simulink model "ex1_500KV_2019a"  (R2023a)
settings: Solver=ode23t  StartTime=0.0  StopTime=1  MaxStep=1e-4  RelTol=1e-3  EnableMultiTasking=on
libraries: spsThreePhaseSourceLib x2, spsDistributedParametersLineLib x2, spsThreePhaseVIMeasurementLib x2, spsThreePhaseFaultLib x1, sps_lib x1
settings Model: SimulationMode=accelerator  Creator=Administrator  LastModifiedBy=Lightrain
settings SolverCC: AlgebraicLoopSolver=TrustRegion
settings DataIOCC: LimitDataPoints=on  SaveFormat=Array  SignalLoggingSaveFormat=ModelDataLogs  ReturnWorkspaceOutputs=off
settings OptimizationCC: ExpressionDepthLimit=2147483647  InitFltsAndDblsToZero=on  LifeSpan=inf
settings DebuggingCC: SaveWithParameterizedLinksMsg=none  UnderspecifiedInitializationDetection=Classic  MergeDetectMultiDrivingBlocksExec=none  SignalResolutionControl=TryResolveAllWithWarning  SolverPrmCheckMsg=warning  MultiTaskDSMMsg=warning  MultiTaskCondExecSysMsg=none  FcnCallInpInsideContextMsg=warning  UnconnectedInputMsg=warning  UnconnectedOutputMsg=warning  UnconnectedLineMsg=warning  StateNameClashWarn=warning  SFUnexpectedBacktrackingDiag=warning  SFNoUnconditionalDefaultTransitionDiag=warning  SFExecutionAtInitializationDiag=none  ArithmeticOperatorsInVariantConditions=warning
settings HardwareCC: ProdBitPerPointer=32  ProdBitPerSizeT=32  ProdBitPerPtrDiffT=32  ProdLargestAtomicFloat=None  ProdIntDivRoundTo=Undefined  ProdEndianess=Unspecified  ProdWordSize=32  ProdHWDeviceType=32-bit Generic
settings ModelReferenceCC: EnableRefExpFcnMdlSchedulingChecks=on  PropagateSignalLabelsOutOfModel=off
settings SFSimCC: SimUseLocalCustomCode=off  CustomCodeUndefinedFunction=UseInterfaceOnly
settings RTWCC: RTWUseLocalCustomCode=off
settings CodeAppCC: StateflowObjectComments=on
settings GRTTargetCC: TargetFcnLib=ansi_tfl_tmw.mat  TargetLangStandard=C89/C90 (ANSI)  CombineOutputUpdateFcns=off  GRTInterface=on
settings ConfigComp: CovMetricSettings=dw  CovSaveCumulativeToWorkspaceVar=on  CovSaveSingleToWorkspaceVar=on  CovExternalEMLEnable=off
settings SimscapeCC: SimscapeNormalizeSystem=off

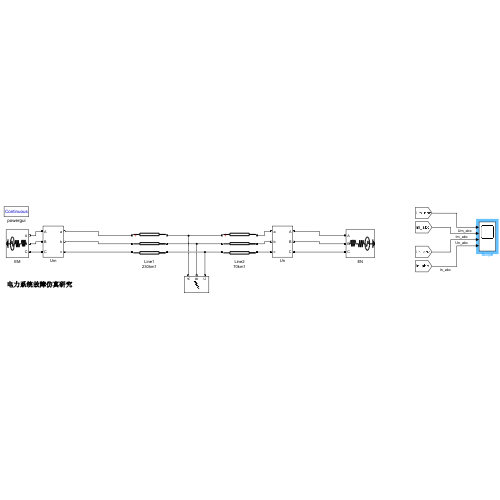
[thumbnail: Simulink's stored preview of the top-level diagram]
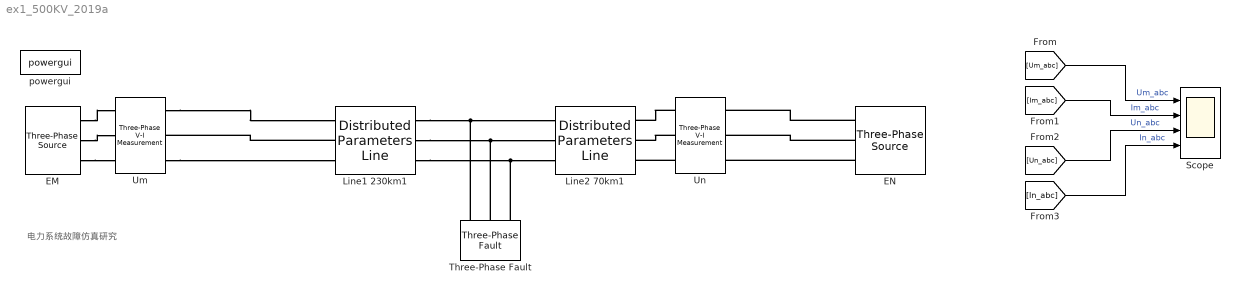
== system ex1_500KV_2019a ==
  note: 电力系统故障仿真研究
  EM : spsThreePhaseSourceLib/Three-Phase Source  InternalConnection=Yg  VoltagePhases=off  Voltage=500e3  PhaseAngle=0  Voltage_phases=[25e3 25e3 25e3]/sqrt(3)  PhaseAngles_phases=[0 -120 +120]  Frequency=50  NonIdealSource=on  SpecifyImpedance=off  Resistance=5.74  Inductance=0.0452  ShortCircuitLevel=100e6  BaseVoltage=25e3  XRratio=7  BusType=swing  Pref=0  Qref=0  Prefabc=[10e3, 10e3, 10e3]  Qrefabc=[0, 0, 0]  Qmin=-inf  Qmax=inf
  EN : spsThreePhaseSourceLib/Three-Phase Source  InternalConnection=Yg  VoltagePhases=off  Voltage=500e3  PhaseAngle=0  Voltage_phases=[25e3 25e3 25e3]/sqrt(3)  PhaseAngles_phases=[0 -120 +120]  Frequency=50  NonIdealSource=on  SpecifyImpedance=off  Resistance=5.74  Inductance=0.0452  ShortCircuitLevel=100e6  BaseVoltage=25e3  XRratio=7  BusType=swing  Pref=0  Qref=0  Prefabc=[10e3, 10e3, 10e3]  Qrefabc=[0, 0, 0]  Qmin=-inf  Qmax=inf
  Line1 230km1 : spsDistributedParametersLineLib/Distributed Parameters Line  Phases=3  Length=230  Frequency=50  Resistance=[ 0.02083 0.1148]  Inductance="[ 0.8984e-3  2.2886e-3]"  Capacitance=[0.0129e-6 5.23e-9]  x1=[2.39996334166363e-10 504386.018905982 504386.018905982;314.159265358979 314.159265358979 314.159265358979;-0.494963403943933 0.274052307116301 -1.2967440196786]  x2=[7.27595761418343e-11 509076.373027704 509076.373027704;314.159265358979 314.159265358979 314.159265358979;2.89160791277272 0.273345233109503 -1.29745109368539]  x3=[1.99350562759694e-12 1909.78676505623 1909.78676505623;314.159265358979 314.159265358979 314.159265358979;0.857163976977022 0.112881553409895 -1.457914773385]  x4=[2.84118265797858e-12 1910.12556335199 1910.12556335199;314.159265358979 314.159265358979 314.159265358979;-1.62338550776208 0.18739970026522 -1.38339662652968]  x5=0.000795726143971656  V1=[2.4e-10 5.044e+05 5.044e+05;314.2 314.2 314.2;-0.495 0.2741 -1.297]  V2=[7.276e-11 5.091e+05 5.091e+05;314.2 314.2 314.2;2.892 0.2733 -1.297]  I1=[1.994e-12 1910 1910;314.2 314.2 314.2;0.8572 0.1129 -1.458]  I2=[2.841e-12 1910 1910;314.2 314.2 314.2;-1.623 0.1874 -1.383]  nHarmo=1  Measurements=Phase-to-ground voltages  Decoupling=off  VsMag0=0  VrMag0=0  VsAngle0=0  VrAngle0=0  IsMag0=0  IrMag0=0  IsAngle0=0  IrAngle0=0
      settings: LibrarySourceBlock=sps_lib/Power Grid Elements/Distributed Parameters Line
  Line2 70km1 : spsDistributedParametersLineLib/Distributed Parameters Line  Phases=3  Length=70  Frequency=50  Resistance=[ 0.02083 0.1148]  Inductance="[ 0.8984e-3  2.2886e-3]"  Capacitance=[0.0129e-6 5.23e-9]  x1=[7.27595761418343e-11 509076.373027704 509076.373027704;314.159265358979 314.159265358979 314.159265358979;3.06551034116721 0.444464764450093 -1.1263315623448]  x2=[4.36557456851006e-11 504385.210793195 504385.210793195;314.159265358979 314.159265358979 314.159265358979;-0.0760823124225862 0.445166778971658 -1.12562954782324]  x3=[4.40693732790997e-12 1928.55532360724 1928.55532360725;314.159265358979 314.159265358979 314.159265358979;-2.04166975891724 0.530127509991258 -1.04066881680363]  x4=[9.99572824572175e-13 1927.6185383434 1927.6185383434;314.159265358979 314.159265358979 314.159265358979;2.32009086489305 0.284472550844726 -1.28632377595018]  x5=0.00024217752207833  V1=[7.276e-11 5.091e+05 5.091e+05;314.2 314.2 314.2;3.066 0.4445 -1.126]  V2=[4.366e-11 5.044e+05 5.044e+05;314.2 314.2 314.2;-0.07608 0.4452 -1.126]  I1=[4.407e-12 1929 1929;314.2 314.2 314.2;-2.042 0.5301 -1.041]  I2=[9.996e-13 1928 1928;314.2 314.2 314.2;2.32 0.2845 -1.286]  nHarmo=1  Measurements=Phase-to-ground voltages  Decoupling=off  VsMag0=0  VrMag0=0  VsAngle0=0  VrAngle0=0  IsMag0=0  IrMag0=0  IsAngle0=0  IrAngle0=0
      settings: LibrarySourceBlock=sps_lib/Power Grid Elements/Distributed Parameters Line
  Scope : Scope  NumInputPorts=4
  Three-Phase Fault : spsThreePhaseFaultLib/Three-Phase Fault  InitialStates=0  FaultA=on  FaultB=off  FaultC=off  GroundFault=on  SwitchTimes=[0.2,1]  External=off  SwitchStatus=NaN  FaultResistance=0.01  GroundResistance=0.00000000001  SnubberResistance=1e6  SnubberCapacitance=inf  Measurements=None
  Um : spsThreePhaseVIMeasurementLib/Three-Phase V-I Measurement  VoltageMeasurement=phase-to-ground  SetLabelV=on  LabelV=Um_abc  Vpu=off  VpuLL=off  CurrentMeasurement=yes  SetLabelI=on  LabelI=Im_abc  Ipu=off  Pbase=100e6  Vbase=500e3  OutputType=Complex  PhasorSimulation=off  PSBequivalent=0
  Un : spsThreePhaseVIMeasurementLib/Three-Phase V-I Measurement  VoltageMeasurement=phase-to-ground  SetLabelV=on  LabelV=Un_abc  Vpu=off  VpuLL=off  CurrentMeasurement=yes  SetLabelI=on  LabelI=In_abc  Ipu=off  Pbase=100e6  Vbase=500e3  OutputType=Complex  PhasorSimulation=off  PSBequivalent=0
  powergui : sps_lib/powergui  SimulationMode=Continuous  SampleTime=0  frequency=50  Iterations=50  frequencyindice=50  Pbase=100e6  ErrMax=1e-4  UnitsV=kV  UnitsW=MW  buscounter=0  FunctionMessages=off  echomessages=off  EnableUseOfTLC=off  CurrentSourceSwitches=off  DisableSnubberDevices=off  DisableRonSwitches=off  DisableVfSwitches=off  DisplayEquations=off  AutomaticDiscreteSolvers=off  SolverType=Tustin  Interpol=off  ExternalGateDelay=off  methode=off  Ts=0  x0status=steady  SPID=off  SwTol=0  HookPort=off  NonlinearTolerance=0  nMaxIteration=15  ContinueOnMaxIteration=off  RestoreLinks=warning  ResistiveCurrentMeasurement=off  Frange=[0:2:500]  Ylog=off  Xlog=on  ShowGrid=off  save=off  variable=ZData  structure=0  ZoomFFT=on  StartTime=0.0  cycles=1  DisplayStyle=1  fundamental=60  FreqAxis=off  MaxFrequency=1000  frequencyindicesteady=1  RmsSteady=2  display=off
  wires:
  [Um_abc] -> Scope/1  "Um_abc"
  [Im_abc] -> Scope/2  "Im_abc"
  [Un_abc] -> Scope/3  "Un_abc"
  [In_abc] -> Scope/4  "In_abc"
  connections:
  Three-Phase Fault/LConn1 -- Line1 230km1/RConn1 -- Line2 70km1/LConn1
  Three-Phase Fault/LConn2 -- Line1 230km1/RConn2 -- Line2 70km1/LConn2
  Three-Phase Fault/LConn3 -- Line1 230km1/RConn3 -- Line2 70km1/LConn3
  EM/RConn3 -- Um/LConn3
  EM/RConn2 -- Um/LConn2
  EM/RConn1 -- Um/LConn1
  Un/RConn3 -- Line2 70km1/RConn3
  Un/RConn2 -- Line2 70km1/RConn2
  Un/RConn1 -- Line2 70km1/RConn1
  Line1 230km1/LConn2 -- Um/RConn2
  Um/RConn3 -- Line1 230km1/LConn3
  Um/RConn1 -- Line1 230km1/LConn1
  EN/RConn3 -- Un/LConn3
  EN/RConn2 -- Un/LConn2
  EN/RConn1 -- Un/LConn1
